simulink model "A1Q5"  (R2021b)
settings: Solver=VariableStepAuto  StartTime=0.0  StopTime=10.0  RelTol=1e-3
libraries: fl_lib x27, nesl_utility x17, spspowerguiLib x1
settings Model: Creator=hansr  LastModifiedBy=hansr

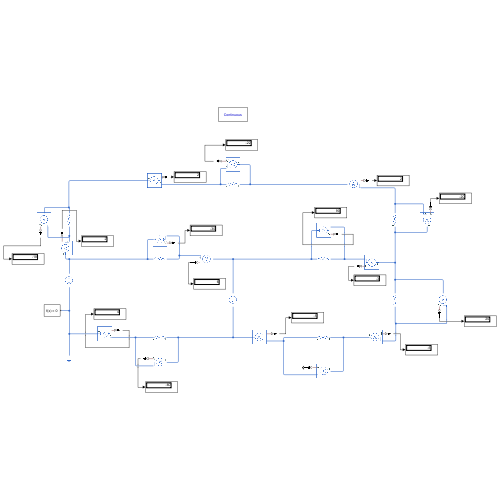
[thumbnail: Simulink's stored preview of the top-level diagram]
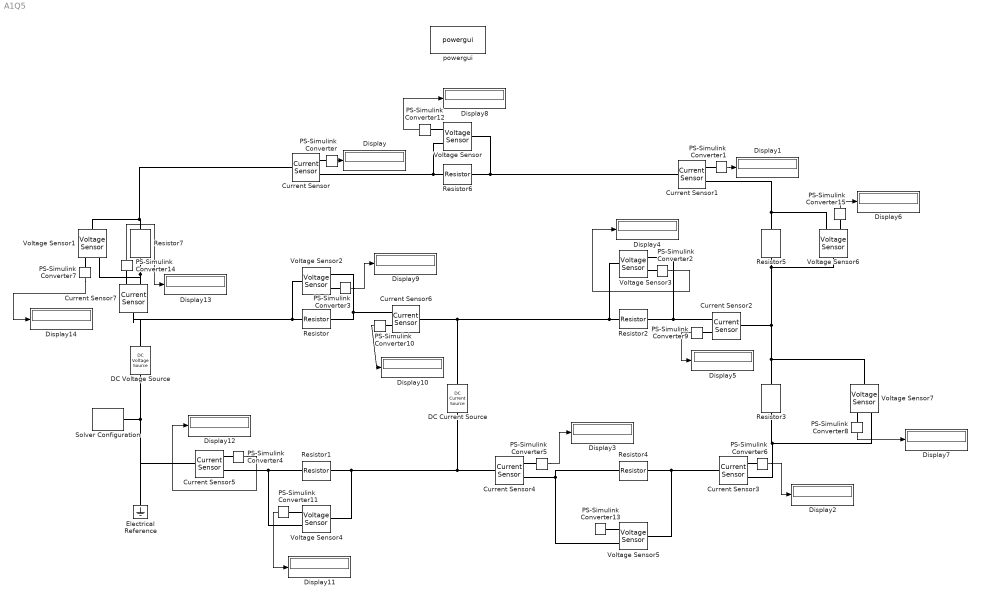
== system A1Q5 ==
  Current Sensor{,1..7} (8 alike) : fl_lib/Electrical/Electrical Sensors/Current Sensor
  DC Current Source : fl_lib/Electrical/Electrical Sources/DC Current Source  i0=-9 A
      settings: SourceProductBaseCode=SS  InternalSimscapePortConfiguration="{\"Bottom\":[],\"Left\":[{\"id\":\"p\",\"label\":\"\",\"type\":\"foundation.electrical.electrical\"}],\"Right\":[{\"id\":\"n\",\"label\":\"\",\"type\":\"foundation.electrical.electrical\"}],\"Top\":[]}"
  DC Voltage Source : fl_lib/Electrical/Electrical Sources/DC Voltage Source  v0=100 V
  Display{,1..14} (15 alike) : Display
  Electrical Reference : fl_lib/Electrical/Electrical Elements/Electrical Reference
  PS-Simulink Converter{,1..15} (16 alike) : nesl_utility/PS-Simulink Converter  PhysicalDomain=network_engine_domain  SubClassName=ps_output  LeftPortType=input  RightPortType=output  PseudoPeriodic=off  Frequencies=[]  Unit=inherit  AffineConversion=off
      settings: SourceProductBaseCode=PW,SS
  Resistor : fl_lib/Electrical/Electrical Elements/Resistor  R=5 Ohm  i_specify=off  i_priority=None  i=0 A  i_nominal_specify=off  i_nominal_unit=A  i_nominal_value=1  v_specify=off  v_priority=None  v=0 V  v_nominal_specify=off  v_nominal_unit=V  v_nominal_value=1
  Resistor1 : fl_lib/Electrical/Electrical Elements/Resistor  R=15 Ohm  i_specify=off  i_priority=None  i=0 A  i_nominal_specify=off  i_nominal_unit=A  i_nominal_value=1  v_specify=off  v_priority=None  v=0 V  v_nominal_specify=off  v_nominal_unit=V  v_nominal_value=1
  Resistor2 : fl_lib/Electrical/Electrical Elements/Resistor  R=30 Ohm  i_specify=off  i_priority=None  i=0 A  i_nominal_specify=off  i_nominal_unit=A  i_nominal_value=1  v_specify=off  v_priority=None  v=0 V  v_nominal_specify=off  v_nominal_unit=V  v_nominal_value=1
  Resistor3 : fl_lib/Electrical/Electrical Elements/Resistor  R=4 Ohm  i_specify=off  i_priority=None  i=0 A  i_nominal_specify=off  i_nominal_unit=A  i_nominal_value=1  v_specify=off  v_priority=None  v=0 V  v_nominal_specify=off  v_nominal_unit=V  v_nominal_value=1
  Resistor4 : fl_lib/Electrical/Electrical Elements/Resistor  R=16 Ohm  i_specify=off  i_priority=None  i=0 A  i_nominal_specify=off  i_nominal_unit=A  i_nominal_value=1  v_specify=off  v_priority=None  v=0 V  v_nominal_specify=off  v_nominal_unit=V  v_nominal_value=1
  Resistor5 : fl_lib/Electrical/Electrical Elements/Resistor  R=10 Ohm  i_specify=off  i_priority=None  i=0 A  i_nominal_specify=off  i_nominal_unit=A  i_nominal_value=1  v_specify=off  v_priority=None  v=0 V  v_nominal_specify=off  v_nominal_unit=V  v_nominal_value=1
  Resistor6 : fl_lib/Electrical/Electrical Elements/Resistor  R=11 Ohm  i_specify=off  i_priority=None  i=0 A  i_nominal_specify=off  i_nominal_unit=A  i_nominal_value=1  v_specify=off  v_priority=None  v=0 V  v_nominal_specify=off  v_nominal_unit=V  v_nominal_value=1
  Resistor7 : fl_lib/Electrical/Electrical Elements/Resistor  R=9 Ohm  i_specify=off  i_priority=None  i=0 A  i_nominal_specify=off  i_nominal_unit=A  i_nominal_value=1  v_specify=off  v_priority=None  v=0 V  v_nominal_specify=off  v_nominal_unit=V  v_nominal_value=1
  Solver Configuration : nesl_utility/Solver Configuration  PhysicalDomain=network_engine_domain  SubClassName=solver  LeftPortType=input  RightPortType=generic  Tones=[]  Harmonics=[]  SimulateNoise=off  Profile=off  UseLocalSampling=off  EnableSwitchedLinearOptims=on  FrequencyDomain=off  UseCCode=off  RelTol=0.001  AbsTol=1e-06  MinStep=1e-09  ToWorkspace=off  RevertToSquareIcSolve=off  NumHomotopyIterations=100  PhasorMode=off  PhasorModeNumHarmonics=1  DoDC=off  ResidualTolerance=1e-09  UseLocalSolver=off  LocalSolverChoice=NE_BACKWARD_EULER_ADVANCER  LocalSolverSampleTime=0.001  DoFixedCost=off  MaxNonlinIter=3  MaxModeIter=2  ComputeImpulses=off  ImpulseIterations=2  LinearAlgebra=auto  EquationFormulation=NE_TIME_EF  DelaysMemoryBudget=1024  AutomaticFiltering=on  FilteringTimeConstant=0.001  PartitionStorageMethod=AS_NEEDED  PartitionMemoryBudget=1024  PartitionMethod=ROBUST
      settings: SourceProductBaseCode=PW,SS
  Voltage Sensor{,1..7} (8 alike) : fl_lib/Electrical/Electrical Sensors/Voltage Sensor
  powergui : spspowerguiLib/powergui  Priority=1  SimulationMode=Continuous  SampleTime=50e-6  frequency=60  Iterations=50  frequencyindice=60  Pbase=100e6  ErrMax=1e-4  UnitsV=kV  UnitsW=MW  buscounter=0  FunctionMessages=off  echomessages=off  EnableUseOfTLC=off  CurrentSourceSwitches=off  DisableSnubberDevices=off  DisableRonSwitches=off  DisableVfSwitches=off  DisplayEquations=off  AutomaticDiscreteSolvers=off  SolverType=Tustin/Backward Euler (TBE)  Interpol=off  ExternalGateDelay=off  methode=off  Ts=100  x0status=blocks  SPID=on  SwTol=0  HookPort=off  NonlinearTolerance=1e-4  nMaxIteration=100  ContinueOnMaxIteration=off  RestoreLinks=warning  ResistiveCurrentMeasurement=off  Frange=[0:2:500]  Ylog=off  Xlog=on  ShowGrid=off  save=off  variable=ZData  structure=0  ZoomFFT=off  StartTime=0.0  cycles=1  DisplayStyle=1  fundamental=60  FreqAxis=off  MaxFrequency=1000  frequencyindicesteady=1  RmsSteady=1  display=off
  wires:
  PS-Simulink Converter/1 -> Display/1
  PS-Simulink Converter1/1 -> Display1/1
  PS-Simulink Converter6/1 -> Display2/1
  PS-Simulink Converter5/1 -> Display3/1
  PS-Simulink Converter2/1 -> Display4/1
  PS-Simulink Converter9/1 -> Display5/1
  PS-Simulink Converter15/1 -> Display6/1
  PS-Simulink Converter8/1 -> Display7/1
  PS-Simulink Converter12/1 -> Display8/1
  PS-Simulink Converter3/1 -> Display9/1
  PS-Simulink Converter10/1 -> Display10/1
  PS-Simulink Converter11/1 -> Display11/1
  PS-Simulink Converter4/1 -> Display12/1
  PS-Simulink Converter14/1 -> Display13/1
  PS-Simulink Converter7/1 -> Display14/1
  connections:
  Resistor/RConn1 -- Current Sensor6/RConn2 -- Voltage Sensor2/RConn2
  DC Voltage Source/RConn1 -- Current Sensor5/LConn1 -- Electrical Reference/LConn1 -- Solver Configuration/RConn1
  Resistor5/LConn1 -- Voltage Sensor6/LConn1 -- Current Sensor2/LConn1 -- Voltage Sensor7/LConn1 -- Resistor3/LConn1
  Voltage Sensor7/RConn2 -- Current Sensor3/RConn2 -- Resistor3/RConn1
  Resistor4/RConn1 -- Current Sensor4/RConn2 -- Voltage Sensor5/RConn2
  Resistor5/RConn1 -- Current Sensor1/RConn2 -- Voltage Sensor6/RConn2
  Resistor6/RConn1 -- Current Sensor/RConn2 -- Voltage Sensor/RConn2
  Voltage Sensor1/LConn1 -- Current Sensor/LConn1 -- Resistor7/LConn1
  Voltage Sensor/LConn1 -- Current Sensor1/LConn1 -- Resistor6/LConn1
  Resistor2/RConn1 -- Current Sensor2/RConn2 -- Voltage Sensor3/RConn2
  Resistor4/LConn1 -- Current Sensor3/LConn1 -- Voltage Sensor5/LConn1
  Voltage Sensor4/LConn1 -- Current Sensor4/LConn1 -- DC Current Source/LConn1 -- Resistor1/LConn1
  Resistor1/RConn1 -- Current Sensor5/RConn2 -- Voltage Sensor4/RConn2
  Voltage Sensor3/LConn1 -- DC Current Source/RConn1 -- Current Sensor6/LConn1 -- Resistor2/LConn1
  Voltage Sensor2/LConn1 -- Current Sensor7/LConn1 -- DC Voltage Source/LConn1 -- Resistor/LConn1
  PS-Simulink Converter/LConn1 -- Current Sensor/RConn1
  PS-Simulink Converter1/LConn1 -- Current Sensor1/RConn1
  PS-Simulink Converter2/LConn1 -- Voltage Sensor3/RConn1
  PS-Simulink Converter3/LConn1 -- Voltage Sensor2/RConn1
  PS-Simulink Converter4/LConn1 -- Current Sensor5/RConn1
  PS-Simulink Converter5/LConn1 -- Current Sensor4/RConn1
  PS-Simulink Converter6/LConn1 -- Current Sensor3/RConn1
  PS-Simulink Converter7/LConn1 -- Voltage Sensor1/RConn1
  PS-Simulink Converter8/LConn1 -- Voltage Sensor7/RConn1
  PS-Simulink Converter9/LConn1 -- Current Sensor2/RConn1
  PS-Simulink Converter10/LConn1 -- Current Sensor6/RConn1
  PS-Simulink Converter11/LConn1 -- Voltage Sensor4/RConn1
  PS-Simulink Converter12/LConn1 -- Voltage Sensor/RConn1
  PS-Simulink Converter13/LConn1 -- Voltage Sensor5/RConn1
  PS-Simulink Converter14/LConn1 -- Current Sensor7/RConn1
  PS-Simulink Converter15/LConn1 -- Voltage Sensor6/RConn1
  Resistor7/RConn1 -- Voltage Sensor1/RConn2 -- Current Sensor7/RConn2
